simulink library "FeatureVersion"  (R2022b)
settings: Solver=VariableStepAuto  StartTime=0.0  StopTime=10.0  RelTol=1e-3
undefined symbols (not defined in the file or in its folder): maskVersionData
libraries: TuneVar x5, CompatHash x2, FeaturePath x1, HandyTextFile x1, RTC x1, StateVar x1
settings Model: Creator=kl13806  LastModifiedBy=kl13806
settings SolverCC: AlgebraicLoopSolver=TrustRegion
settings DebuggingCC: UnconnectedInputMsg=warning  UnconnectedOutputMsg=warning  UnconnectedLineMsg=warning  SFMachineParentedDataDiag=warning  ArithmeticOperatorsInVariantConditions=warning
settings ModelReferenceCC: EnableRefExpFcnMdlSchedulingChecks=on
settings SFSimCC: SimUseLocalCustomCode=off  CustomCodeUndefinedFunction=UseInterfaceOnly
settings RTWCC: RTWUseLocalCustomCode=off  DLArmComputeVersion=19.05

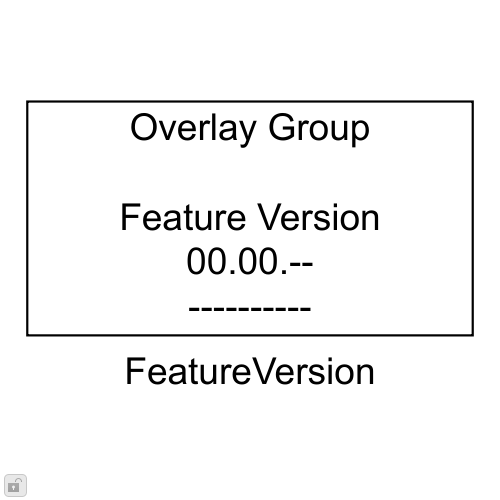
[thumbnail: Simulink's stored preview of the top-level diagram]
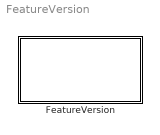
== system FeatureVersion ==
  FeatureVersion : Subsystem  mask(Talaria Feature Version){Major=0, Minor=0, Patch=AA, String=, BankNumber=0, IncludeCompatHash=DefaultNoCompatHash, IncludeRtc=DefaultUseTspOnly, TriggerInit=[]}
      mask prompts: BankNumber "Target memory bank number:"; IncludeCompatHash "Include legacy COMPAT_HASH retrieval"; IncludeRtc "Include legacy read-only RTC interface"; TriggerInit "Hidden: dialog open, MoveFcn"
      mask help:
      | This block contains version information to be retrieved by control code. Enter the feature version information below which will be built statically into the binary code image.
      | This block also encapsulates tuning data versions which are loaded into DSP memory along with other tuning data.
      mask init:
      | [ok,groupPath,maskVersionData,displayVersion,displayString] = FeatureVersionMask.DoInit(gcbh,Major,Minor,Patch,String);
      settings: MoveFcn=FeatureVersionMask.CB_TriggerInit(gcbh);
      mask Help: There is a need to retain version information for the current tuning database within the feature. Before Talaria, the micro retrieved the version information directly from the DB when needed. But for our PSS implementations, we do not have a micro to manage these version requests.
      mask TypeOptions BankNumber: TuningDataSetVersion/BankNumber | TuningBuildDateTime/BankNumber | TuningBuildHost/BankNumber | TuningBuildUser/BankNumber | TuningBuildCartype/BankNumber
      mask TypeOptions IncludeCompatHash: CompatHash/LabelModeActiveChoice
      mask TypeOptions IncludeRtc: LegacyRtc/LabelModeActiveChoice
      mask Callback TriggerInit: FeatureVersionMask.CB_TriggerInit(gcbh);
      mask DialogControl FeatureVersionGroup Prompt: Feature Version Settings (design time)
      mask DialogControl TuningVersionGroup Prompt: Tuning Version Settings (tuning)
      mask DialogControl ErrorContainer Prompt: Error Messages
      mask Display:
      | % retrieve the block's pixel size
      | pos = get(gcbh,'position');
      | bw = pos(3) - pos(1);
      | bh = pos(4) - pos(2);
      | 
      | % show version information or an X
      | if (exist('ok','var') && ok)
      |    iconText=sprintf('%s\n\nFeature Version\n%s\n%s', ...
      |              groupPath,displayVersion,displayString);
      |    disp(iconText);
      | else
      | 	tx=bw*0.03;
      | 	ty=bh*0.03;
      | 	patch([0 tx bw bw-tx], [ty 0 bh-ty bh], [1 0 0]);
      | 	patch([0 bw-tx bw tx], [bh-ty 0 ty bh], [1 0 0]);
      | end

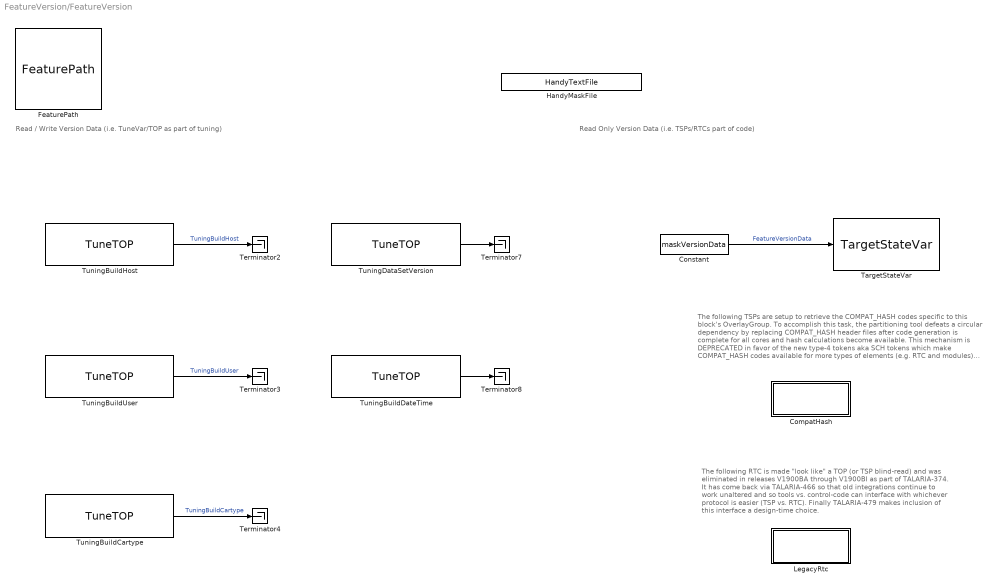
== system FeatureVersion/FeatureVersion ==
  note: The following TSPs are setup to retrieve the COMPAT_HASH codes specific
      | to this block's OverlayGroup. To accomplish this task, the partitioning tool
      | defeats a circular dependency by replacing COMPAT_HASH header files
      | after code generation is complete for all cores and hash calculations become
      | available. This mechanism is DEPRECATED in favor of the new type-4 tokens
      | aka SCH tokens which make COMPAT_HASH codes available for more
      | types of elements (e.g. RTC and modules) and use static unchanging token IDs.
  note: Read Only Version Data (i.e. TSPs/RTCs part of code)
  note: Read / Write Version Data (i.e. TuneVar/TOP as part of tuning)
  note: The following RTC is made "look like" a TOP (or TSP blind-read)
      | and was eliminated in releases V1900BA through V1900BI as part
      | of TALARIA-374. It has come back via TALARIA-466 so that old
      | integrations continue to work unaltered and so tools vs. control-code
      | can interface with whichever protocol is easier (TSP vs. RTC). Finally
      | TALARIA-479 makes inclusion of this interface a design-time choice.
  CompatHash : Subsystem  Variant=on  VariantControlMode=label  LabelModeActiveChoice=DefaultNoCompatHash
  Constant : Constant  Value=maskVersionData
  FeaturePath : FeaturePath/FeaturePath  FeatureName=Feature  IsGroup=off  GroupNumber=-1  IsModule=off  TriggerInit=[-70 -1046 45 -939]
      settings: SourceProductName=Bose Talaria
  HandyMaskFile : HandyTextFile/HandyTextFile  TemplateSource=Mask  FileSuffix=Init  OpenDialogOnLoad=off  UseThisBlockName=off  TheDefaultText=|  ShowInLibBrowser=on
      | % $(FILENAME) Setup model parameters for each "Init" callback (e.g. update diagram)
      | sample_rate_in_hertz = 44100;
      | frame_size = 32;
      | sysin_channel_count = 2;
      settings: SourceProductName=Bose Talaria
  LegacyRtc : Subsystem  Variant=on  VariantControlMode=label  LabelModeActiveChoice=DefaultUseTspOnly
  TargetStateVar : StateVar/TargetStateVar  TriggerInit=[1015 -794 1155 -726]  TspName=Version  StateName=Version  UseSameName=on  IfdefMacro='CAPTURE_CONSTANT_TSPS'
      settings: SourceProductName=Bose Talaria
  Terminator{2..4,7..8} (5 alike) : Terminator
  TuningBuildCartype : TuneVar/TuneTOP  TriggerInit=[-30 -428 140 -372]  TopName=TuningBuildCartype  TuneName=TuningBuildCartype  DataType=Inherit: Same as input  TunabilityNumber=1  MinValue=[]  MaxValue=[]  BankNumber=BankNumber  PreOverlay=false  PostOverlay=false  UseSameName=on  MaskValue=repmat(char(0),1,16)
      settings: SourceProductName=Bose Talaria
  TuningBuildDateTime : TuneVar/TuneTOP  TriggerInit=[350 -613 520 -557]  TopName=TuningBuildDateTime  TuneName=TuningBuildDateTime  DataType=uint8  TunabilityNumber=1  MinValue=[]  MaxValue=[]  BankNumber=BankNumber  PreOverlay=false  PostOverlay=false  UseSameName=on  MaskValue=uint8(zeros(1,6))
      settings: SourceProductName=Bose Talaria
  TuningBuildHost : TuneVar/TuneTOP  TriggerInit=[-30 -788 140 -732]  TopName=TuningBuildHost  TuneName=TuningBuildHost  DataType=Inherit: Same as input  TunabilityNumber=1  MinValue=[]  MaxValue=[]  BankNumber=BankNumber  PreOverlay=false  PostOverlay=false  UseSameName=on  MaskValue=repmat(char(0),1,16)
      settings: SourceProductName=Bose Talaria
  TuningBuildUser : TuneVar/TuneTOP  TriggerInit=[-30 -613 140 -557]  TopName=TuningBuildUser  TuneName=TuningBuildUser  DataType=Inherit: Same as input  TunabilityNumber=1  MinValue=[]  MaxValue=[]  BankNumber=BankNumber  PreOverlay=false  PostOverlay=false  UseSameName=on  MaskValue=repmat(char(0),1,12)
      settings: SourceProductName=Bose Talaria
  TuningDataSetVersion : TuneVar/TuneTOP  TriggerInit=[350 -788 520 -732]  TopName=TuningDataSetVersion  TuneName=TuningDataSetVersion  DataType=uint8  TunabilityNumber=1  MinValue=[]  MaxValue=[]  BankNumber=BankNumber  PreOverlay=false  PostOverlay=false  UseSameName=on  MaskValue=uint8(zeros(1,14))
      settings: SourceProductName=Bose Talaria
  wires:
  TuningDataSetVersion/1 -> Terminator7/1
  TuningBuildDateTime/1 -> Terminator8/1
  TuningBuildHost/1 -> Terminator2/1  "TuningBuildHost"
  TuningBuildUser/1 -> Terminator3/1  "TuningBuildUser"
  TuningBuildCartype/1 -> Terminator4/1  "TuningBuildCartype"
  Constant/1 -> TargetStateVar/1  "FeatureVersionData"

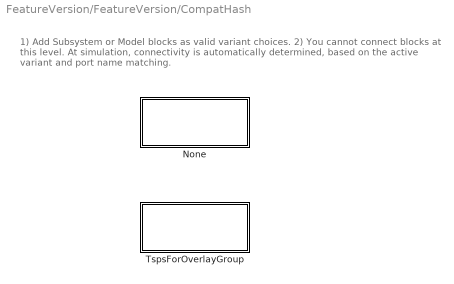
== system FeatureVersion/FeatureVersion/CompatHash ==
  note: 1) Add Subsystem or Model blocks as valid variant choices.
      | 2) You cannot connect blocks at this level. At simulation, connectivity is automatically
      | determined, based on the active variant and port name matching.
  None : Subsystem  VariantControl=DefaultNoCompatHash
  TspsForOverlayGroup : Subsystem  VariantControl=LegacyCompatHash

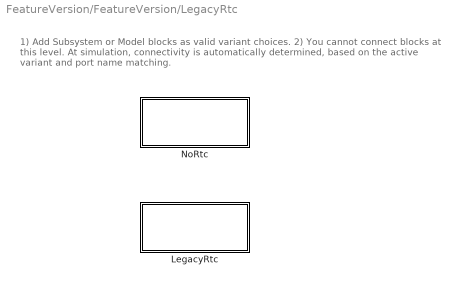
== system FeatureVersion/FeatureVersion/LegacyRtc ==
  note: 1) Add Subsystem or Model blocks as valid variant choices.
      | 2) You cannot connect blocks at this level. At simulation, connectivity is automatically
      | determined, based on the active variant and port name matching.
  LegacyRtc : Subsystem  VariantControl=AlsoIncludeRtc
  NoRtc : Subsystem  VariantControl=DefaultUseTspOnly

== system FeatureVersion/FeatureVersion/CompatHash/None ==

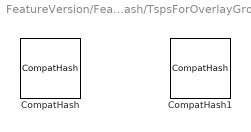
== system FeatureVersion/FeatureVersion/CompatHash/TspsForOverlayGroup ==
  CompatHash : CompatHash/CompatHash  CompatType=TOP: COMPAT code for Target Overlay Parameter tokens
  CompatHash1 : CompatHash/CompatHash  CompatType=TSP: COMPAT code for Target State Probe tokens

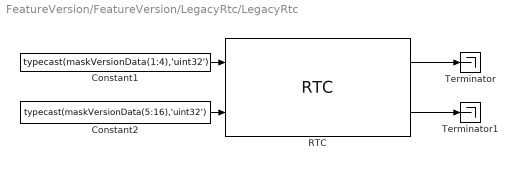
== system FeatureVersion/FeatureVersion/LegacyRtc/LegacyRtc ==
  Constant1 : Constant  Value=typecast(maskVersionData(1:4),'uint32')
  Constant2 : Constant  Value=typecast(maskVersionData(5:16),'uint32')
  RTC : RTC/RTC  REQ_Priority=RTC_Mask.NormalPriority  RequestAtInit=off  EnableRequest=off  REQElemName1=unusedOffset  REQElemType1=uint32  REQElemWidth1=1  REQElemInitial1=[]  REQElemName2=unusedByteCount  REQElemType2=uint32  REQElemWidth2=1  REQElemInitial2=[]  REQElemType3=uint32  REQElemWidth3=1  REQElemInitial3=[]  REQElemType4=uint32  REQElemWidth4=1  REQElemInitial4=[]  REQElemType5=uint32  REQElemWidth5=1  REQElemInitial5=[]  REQElemType6=uint32  REQElemWidth6=1  REQElemInitial6=[]  REQElemType7=uint32  REQElemWidth7=1  REQElemInitial7=[]  REQElemType8=uint32  REQElemWidth8=1  REQElemInitial8=[]  REQElemType9=uint32  REQElemWidth9=1  REQElemInitial9=[]  REQElemType10=uint32  REQElemWidth10=1  REQElemInitial10=[]  EnableResponse=on  EnableRSP_StatusIn=off  RSPElemName1=versionData  RSPElemType1=uint32  RSPElemWidth1=1  RSPElemName2=versionString  RSPElemType2=uint32  RSPElemWidth2=3  RSPElemType3=uint32  RSPElemWidth3=1  RSPElemType4=uint32  RSPElemWidth4=1  RSPElemType5=uint32  RSPElemWidth5=1  RSPElemType6=uint32  RSPElemWidth6=1  RSPElemType7=uint32  RSPElemWidth7=1  RSPElemType8=uint32  RSPElemWidth8=1  RSPElemType9=uint32  RSPElemWidth9=1  RSPElemType10=uint32  RSPElemWidth10=1  EnableNotification=off  EnableNTF_PrepTrig=off  NTFElemType1=uint32  NTFElemWidth1=1  NTFElemType2=uint32  NTFElemWidth2=1  NTFElemType3=uint32  NTFElemWidth3=1  NTFElemType4=uint32  NTFElemWidth4=1  NTFElemType5=uint32  NTFElemWidth5=1  NTFElemType6=uint32  NTFElemWidth6=1  NTFElemType7=uint32  NTFElemWidth7=1  NTFElemType8=uint32  NTFElemWidth8=1  NTFElemType9=uint32  NTFElemWidth9=1  NTFElemType10=uint32  NTFElemWidth10=1  MaskMessageName=Version
      settings: SourceProductName=Bose Talaria
  Terminator : Terminator
  Terminator1 : Terminator
  wires:
  Constant2/1 -> RTC/2
  Constant1/1 -> RTC/1
  RTC/2 -> Terminator1/1
  RTC/1 -> Terminator/1

== system FeatureVersion/FeatureVersion/LegacyRtc/NoRtc ==
